simulink model "vrmemb1"  (Simulink 7.4)
settings: Solver=VariableStepDiscrete  StartTime=0.0  StopTime=Inf  RelTol=1e-3
PostLoadFcn:
  | vrmemb1_callbacks PostLoad;
libraries: simulink x5, vrlib x1
Description:
  | Rotating Membrane
  | 
  | The vrmemb1 example is similar to the vrmemb example, but this time the associated
  | virtual world is driven from a Simulink(R) model.
settings Model: Creator=Danek  LastModifiedBy=Houska  CovMetricSettings=d  ExtModeTrigMode=oneshot  ExtModeArmWhenConnect=off  ExtModeAutoUpdateStatusClock=off
settings DataIOCC: LimitDataPoints=off  SaveOutput=off  SaveTime=off  SignalLoggingName=logsOut
settings OptimizationCC: BlockReduction=off  BooleanDataType=off  InlineInvariantSignals=on  InitFltsAndDblsToZero=on
settings DebuggingCC: CheckExecutionContextPreStartOutputMsg=on  CheckExecutionContextRuntimeOutputMsg=on  SignalResolutionControl=TryResolveAllWithWarning  SolverPrmCheckMsg=none  MultiTaskDSMMsg=warning  MultiTaskCondExecSysMsg=none  StrictBusMsg=None
settings HardwareCC: TargetUnknown=on
settings ModelReferenceCC: UpdateModelReferenceTargets=IfOutOfDate
settings SFSimCC: SimGenerateEmlReport=off
settings RTWCC: IncludeERTFirstTime=on
settings GRTTargetCC: TargetFcnLib=ansi_tfl_tmw.mat

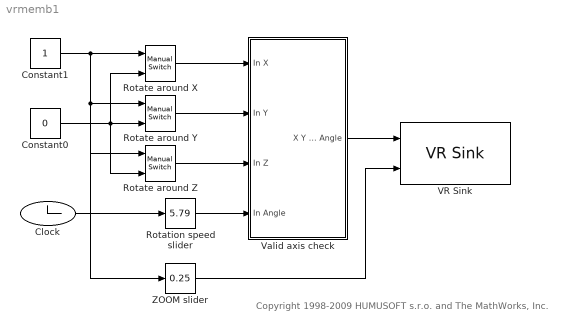
== system vrmemb1 ==
  note: Copyright 1998-2009 HUMUSOFT s.r.o. and The MathWorks, Inc.
  Clock : Clock
  Constant0 : Constant  Value=0  OutDataType=sfix(16)  OutScaling=2^0
  Constant1 : Constant  OutDataType=sfix(16)  OutScaling=2^0
  Rotate around X : simulink/Signal Routing/Manual Switch  SystemSampleTime=-1  sw=0  action=0  varsize=off
  Rotate around Y : simulink/Signal Routing/Manual Switch  SystemSampleTime=-1  sw=0  action=0  varsize=off
  Rotate around Z : simulink/Signal Routing/Manual Switch  SystemSampleTime=-1  sw=1  action=0  varsize=off
  Rotation speed slider : simulink/Math Operations/Slider Gain  SystemSampleTime=-1  low=0  gain=5.79  high=10
  VR Sink : vrlib/VR Sink  InstantiateOnLoad=on  SampleTime=0.01  ViewEnable=on  RemoteChange=off  RemoteView=off  FieldsWritten=Membrane.rotation.4.1.double#View1.fieldOfView.1.1.double  WorldFileName=membrane.wrl  AutoView=on  VideoDimensions=[]  FigureProperties="{'Position', 'Name', 'Viewpoint', 'CameraBound', 'CameraDirection', 'CameraPosition', 'CameraUpVector', 'ZoomFactor', 'Antialiasing', 'Headlight', 'Lighting', 'NavPanel', 'StatusBar', 'ToolBar', 'Textures', 'Transparency', 'Wireframe', 'NavZones', 'NavMode', 'NavSpeed', 'Record2DCompressMethod', 'Record2DCompressQuality', 'Record2D', 'Record2DFileName', 'Record2DFPS'; [5.0000000000000000e+000  9.2000000000000000e+001  5.7600000000000000e+002  3.8000000000000000e+002], 'VRML MATLAB Membrane', 'Original view', 'on', [0.0000000000000000e+000  0.0000000000000000e+000 -1.0000000000000000e+000], [0.0000000000000000e+000  0.0000000000000000e+000  0.0000000000000000e+000], [0.0000000000000000e+000  1.0000000000000000e+000  0.0000000000000000e+000], [1.0000000000000000e+000], 'off', 'off', 'on', 'halfbar', 'on', 'on', 'on', 'on', 'off', 'off', 'examine', 'normal', 'auto', [7.5000000000000000e+001], 'off', '%f_anim_%n.avi', [1.5000000000000000e+001]}"
  Valid axis check : Subsystem  Description=This block is used for eliminating the [ 0 0 0 X ] combination of inputs, which would result in undefined rotation.
  ZOOM slider : simulink/Math Operations/Slider Gain  Description=Use this slider to ZOOM the scene - controls the fieldOfView parameter of View1  SystemSampleTime=-1  low=0.25  gain=0.25  high=0.8
  wires:
  Constant1/1 -> Rotate around X/1, Rotate around Y/1, Rotate around Z/1, ZOOM slider/1
  Constant0/1 -> Rotate around X/2, Rotate around Y/2, Rotate around Z/2
  Rotate around X/1 -> Valid axis check/1(In X)
  Rotate around Y/1 -> Valid axis check/2(In Y)
  Rotate around Z/1 -> Valid axis check/3(In Z)
  Rotation speed slider/1 -> Valid axis check/4(In Angle)
  Clock/1 -> Rotation speed slider/1
  ZOOM slider/1 -> VR Sink/2
  Valid axis check/1(X Y Z Angle) -> VR Sink/1

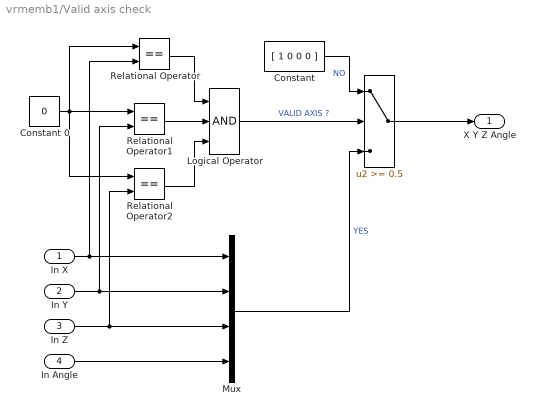
== system vrmemb1/Valid axis check ==
  In X : Inport  OutDataType=sfix(16)  OutScaling=2^0
  In Y : Inport  Port=2  OutDataType=sfix(16)  OutScaling=2^0
  In Z : Inport  Port=3  OutDataType=sfix(16)  OutScaling=2^0
  In Angle : Inport  Port=4  OutDataType=sfix(16)  OutScaling=2^0
  " " : Switch  Threshold=0.5  OutDataType=sfix(16)  OutScaling=2^0  InputSameDT=on
  Constant : Constant  Value=[ 1 0 0 0 ]  OutDataType=sfix(16)  OutScaling=2^0
  Constant 0 : Constant  Value=0  OutDataType=sfix(16)  OutScaling=2^0
  Logical Operator : Logic  Inputs=3
  Mux : Mux
  Relational Operator : RelationalOperator  Operator===  InputSameDT=on
  Relational Operator1 : RelationalOperator  Operator===  InputSameDT=on
  Relational Operator2 : RelationalOperator  Operator===  InputSameDT=on
  X Y Z Angle : Outport  OutDataType=sfix(16)  OutScaling=2^0
  wires:
  Constant 0/1 -> Relational Operator1/1, Relational Operator2/1, Relational Operator/1
  Relational Operator1/1 -> Logical Operator/2
  Relational Operator2/1 -> Logical Operator/3
  Relational Operator/1 -> Logical Operator/1
  In Z/1 -> Relational Operator2/2, Mux/3
  In Y/1 -> Relational Operator1/2, Mux/2
  In X/1 -> Relational Operator/2, Mux/1
  Mux/1 -> " "/3  "YES"
  Logical Operator/1 -> " "/2  "VALID AXIS ?"
  In Angle/1 -> Mux/4
  " "/1 -> X Y Z Angle/1
  Constant/1 -> " "/1  "NO"
